simulink model "lab_modulation_fm"  (R2022a)
settings: Solver=VariableStepAuto  StartTime=0.0  StopTime=10.0  RelTol=1e-3
libraries: dspmathops x1, commanapbnd3 x1, dspfdesign x1
settings Model: Creator=salgi  LastModifiedBy=salgi

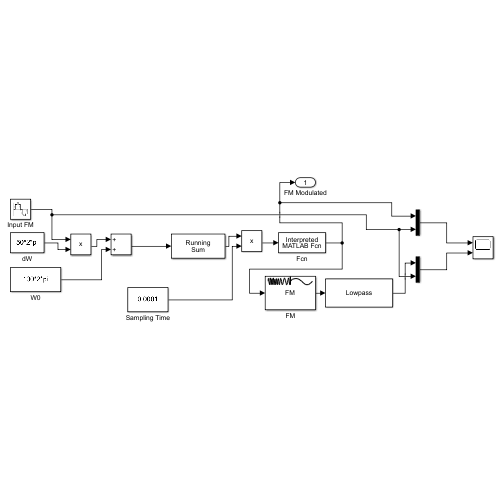
[thumbnail: Simulink's stored preview of the top-level diagram]
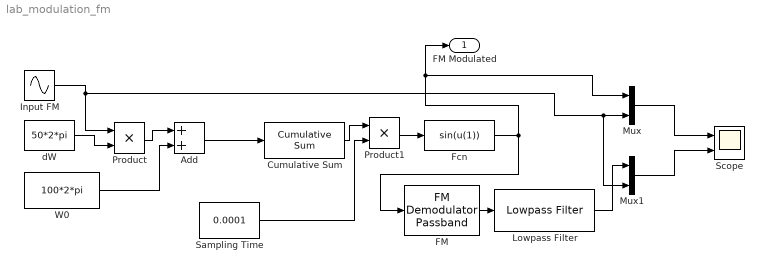
== system lab_modulation_fm ==
  Add : Sum
  Cumulative Sum : dspmathops/Cumulative Sum  dim=Channels (running sum)  reset_popup=None  roundingMode=Floor  overflowMode=off  outputDataTypeStr=Inherit: Same as accumulator  outputMin=[]  outputMax=[]  outputLastDataTypeStr=Inherit: Same as accumulator
  FM : commanapbnd3/FM Demodulator Passband  Fc=100  Ph=0  Kc=50  Ho=100
      settings: SourceProductBaseCode=CM
  Fcn : MATLABFcn  MATLABFcn=sin(u(1))
  Input FM : Sin  Frequency=4*pi  SampleTime=0.0001
  Lowpass Filter : dspfdesign/Lowpass Filter  FilterType=FIR  DesignForMinimumOrder=on  FilterOrder=50  PassbandFrequency=0.1  StopbandFrequency=100  PassbandRipple=0.1  StopbandAttenuation=80  InheritSampleRate=on  SampleRate=44100  SimulateUsing=Interpreted execution  roundingMode=Floor  coeffsDataTypeStr=fixdt(1,16)
  Mux : Mux  Inputs=2
  Mux1 : Mux  Inputs=2
  Product : Product
  Product1 : Product
  Sampling Time : Constant  Value=0.0001
  Scope : Scope  NumInputPorts=2
  W0 : Constant  Value=100*2*pi
  dW : Constant  Value=50*2*pi
  FM Modulated : Outport
  wires:
  Mux1/1 -> Scope/2
  Mux/1 -> Scope/1
  Lowpass Filter/1 -> Mux1/1
  Fcn/1 -> Mux/1, FM Modulated/1, FM/1
  Sampling Time/1 -> Product1/2
  Input FM/1 -> Mux1/2, Mux/2, Product/1
  FM/1 -> Lowpass Filter/1
  Product/1 -> Add/1
  dW/1 -> Product/2
  Cumulative Sum/1 -> Product1/1
  Add/1 -> Cumulative Sum/1
  Product1/1 -> Fcn/1
  W0/1 -> Add/2
